simulink model "Clutch"  (R2020b)
settings: Solver=VariableStepAuto  StartTime=0.0  StopTime=10.0  RelTol=1e-3
settings Model: Creator=Sourav Kumar  LastModifiedBy=Sourav Kumar

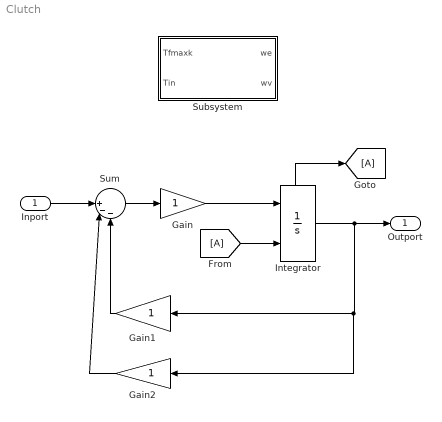
== system Clutch ==
  Inport : Inport
  Gain : Gain
  Gain1 : Gain
  Gain2 : Gain
  Integrator : Integrator  InitialConditionSource=external  ShowStatePort=on
  Subsystem : Subsystem
  Sum : Sum  Inputs=||+--
  Outport : Outport
  wires:
  [A] -> Integrator/2
  Gain1/1 -> Sum/3
  Gain2/1 -> Sum/2
  Inport/1 -> Sum/1
  Sum/1 -> Gain/1
  Gain/1 -> Integrator/1
  Integrator/State -> [A]
  Integrator/1 -> Gain2/1, Gain1/1, Outport/1

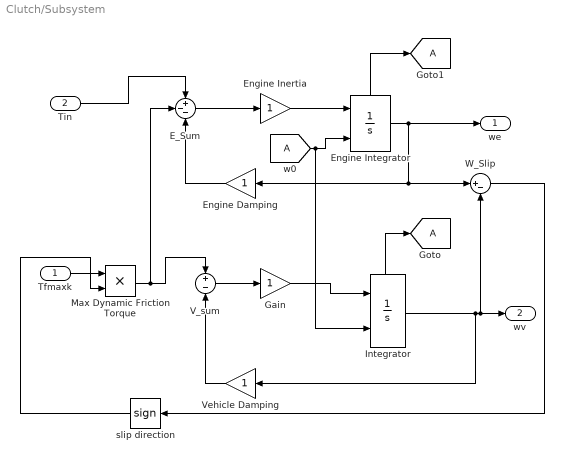
== system Clutch/Subsystem ==
  Tfmaxk : Inport
  Tin : Inport  Port=2
  E_Sum : Sum  Inputs=+--
  Engine Damping : Gain
  Engine Inertia : Gain
  Engine Integrator : Integrator  InitialConditionSource=external  ShowStatePort=on
  Gain : Gain
  Integrator : Integrator  InitialConditionSource=external  ShowStatePort=on
  Max Dynamic Friction Torque : Product
  V_sum : Sum  Inputs=+-
  Vehicle Damping : Gain
  W_Slip : Sum  Inputs=|+-  InputSameDT=on  SaturateOnIntegerOverflow=on  OutDataTypeStr=Inherit: Same as first input
  slip direction : Signum
  we : Outport
  wv : Outport  Port=2
  tag scope: A=global
  wires:
  slip direction/1 -> Max Dynamic Friction Torque/2
  Integrator/1 -> wv/1, W_Slip/2, Vehicle Damping/1
  Tin/1 -> E_Sum/1
  Engine Damping/1 -> E_Sum/3
  Gain/1 -> Integrator/1
  Engine Integrator/1 -> we/1, Engine Damping/1, W_Slip/1
  Max Dynamic Friction Torque/1 -> E_Sum/2, V_sum/1
  Engine Integrator/State -> [A]
  E_Sum/1 -> Engine Inertia/1
  W_Slip/1 -> slip direction/1
  V_sum/1 -> Gain/1
  Tfmaxk/1 -> Max Dynamic Friction Torque/1
  Vehicle Damping/1 -> V_sum/2
  Engine Inertia/1 -> Engine Integrator/1
  Integrator/State -> [A]
  [A] -> Integrator/2, Engine Integrator/2
